simulink model "Feedforward_Control"  (R2025b)
settings: Solver=FixedStepAuto  StartTime=0.0  StopTime=tspan  FixedStep=dt_sim  RelTol=rel_tol  AbsTol=abs_tol
undefined symbols (not defined in the file): battery_voltage, mission_file, mode_id
settings Model: Creator=koryh  LastModifiedBy=matthewlin

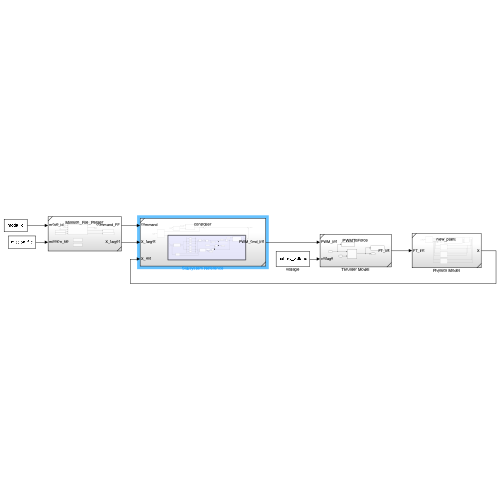
[thumbnail: Simulink's stored preview of the top-level diagram]
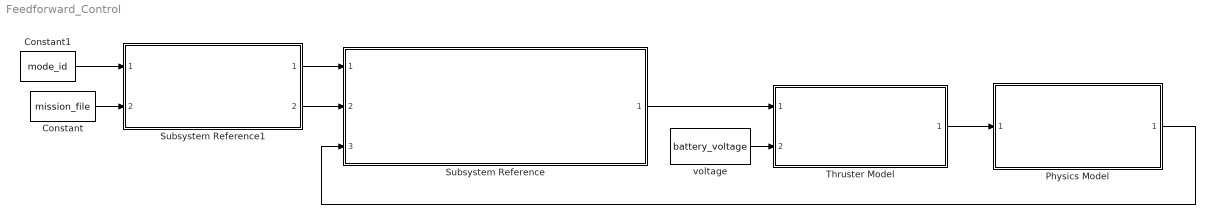
== system Feedforward_Control ==
  Constant : Constant  Value=mission_file
  Constant1 : Constant  Value=mode_id
  Physics Model : Subsystem  ReferencedSubsystem=new_plant
  Subsystem Reference : Subsystem  ReferencedSubsystem=controller
  Subsystem Reference1 : Subsystem  ReferencedSubsystem=Mission_File_Parser
  Thruster Model : Subsystem  ReferencedSubsystem=PWMToForce
  voltage : Constant  Value=battery_voltage
  wires:
  Thruster Model/1 -> Physics Model/1
  voltage/1 -> Thruster Model/2
  Constant/1 -> Subsystem Reference1/2
  Constant1/1 -> Subsystem Reference1/1
  Subsystem Reference1/2 -> Subsystem Reference/2
  Physics Model/1 -> Subsystem Reference/3
  Subsystem Reference/1 -> Thruster Model/1
  Subsystem Reference1/1 -> Subsystem Reference/1
